simulink model "lab3_s"  (R2022b)
settings: Solver=VariableStepAuto  StartTime=0.0  StopTime=czas_symulacji  RelTol=1e-3
values from neighbouring files (symbols this model uses):
  a0 = 5    [lab3.m]
  a1 = 7    [lab3.m]
  b = 7    [lab3.m]
  du = 1    [lab3.m]
  t0 = 10    [lab3.m]
  u0 = 0    [lab3.m]
  x0 = b*u0/a0    (= 0)    [lab3.m]
settings Model: Creator=Dawid  LastModifiedBy=Dawid
settings DataIOCC: ReturnWorkspaceOutputs=off

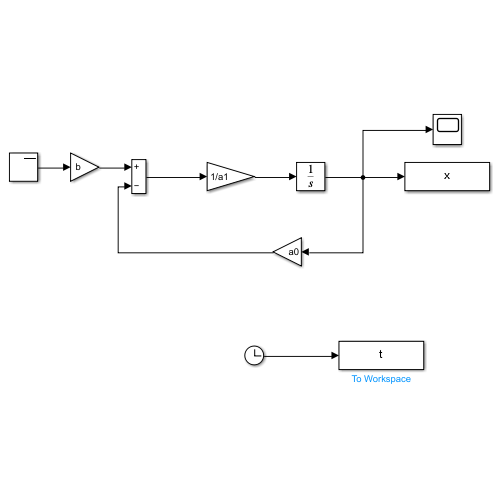
[thumbnail: Simulink's stored preview of the top-level diagram]
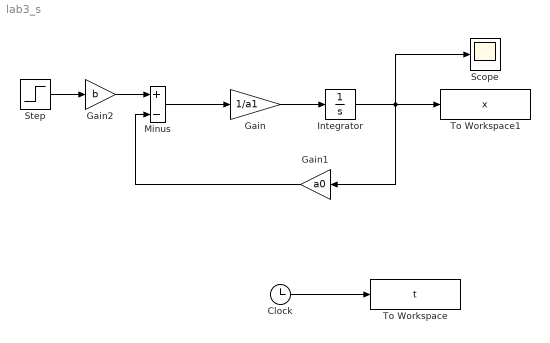
== system lab3_s ==
  Clock : Clock
  Gain : Gain  Gain=1/a1
  Gain1 : Gain  Gain=a0
  Gain2 : Gain  Gain=b
  Integrator : Integrator  InitialCondition=x0
  Minus : Sum  Inputs=+-
  Scope : Scope
  Step : Step  Time=t0  Before=u0  After=u0+du  SampleTime=0
  To Workspace : ToWorkspace  VariableName=t  SaveFormat=Timeseries  SampleTime=-1
  To Workspace1 : ToWorkspace  VariableName=x  SampleTime=-1
  wires:
  Clock/1 -> To Workspace/1
  Integrator/1 -> Scope/1, To Workspace1/1, Gain1/1
  Gain/1 -> Integrator/1
  Gain1/1 -> Minus/2
  Minus/1 -> Gain/1
  Step/1 -> Gain2/1
  Gain2/1 -> Minus/1
